simulink model "model_2springs_with_PSnum"  (R2023a)
settings: Solver=ode4  StartTime=0.0  StopTime=model.tmax  FixedStep=model.dt  RelTol=1e-3
values from neighbouring files (symbols this model uses):
  element : value not decoded    [Elem9_L5_NL4.sldd]
  model : value not decoded    [Elem9_L5_NL4.sldd]
settings Model: DataDictionary=model_2springs.sldd  Creator=glenn  LastModifiedBy=glenn
settings DataIOCC: SaveState=on
settings DebuggingCC: AlgebraicLoopMsg=none

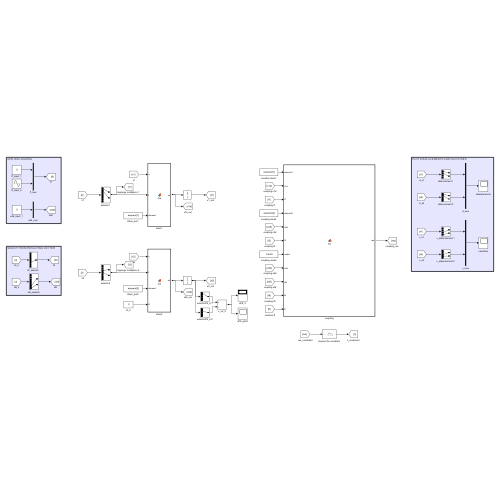
[thumbnail: Simulink's stored preview of the top-level diagram]
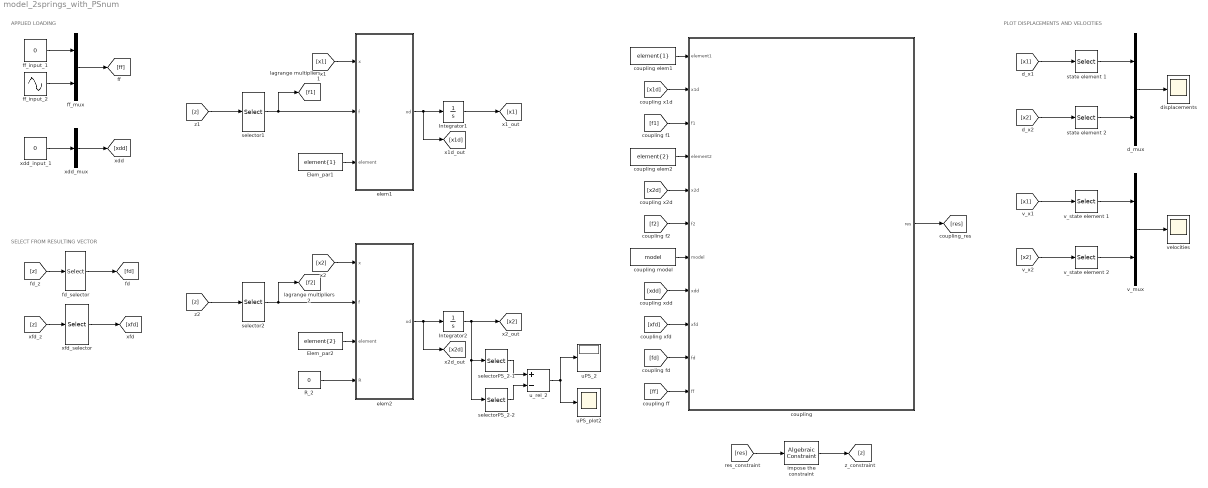
== system model_2springs_with_PSnum ==
  note: APPLIED LOADING
  note: SELECT FROM RESULTING VECTOR
  note: PLOT DISPLACEMENTS AND VELOCITIES
  Elem_par1 : Constant  Value=element{1}  OutDataTypeStr=Bus: ePar1
  Elem_par2 : Constant  Value=element{2}  OutDataTypeStr=Bus: ePar2
  Integrator1 : Integrator  InitialCondition=zeros(4,1)
  Integrator2 : Integrator  InitialCondition=zeros(5,1)
  R_2 : Constant  Value=0
  coupling : MATLAB Function  TreatAsAtomicUnit=on
  coupling elem1 : Constant  Value=element{1}  OutDataTypeStr=Bus: ePar1
  coupling elem2 : Constant  Value=element{2}  OutDataTypeStr=Bus: ePar2
  coupling model : Constant  Value=model  OutDataTypeStr=Bus: mPar
  d_mux : Mux  Inputs=2
  displacements : Scope
  elem1 : MATLAB Function  TreatAsAtomicUnit=on
  elem2 : MATLAB Function  TreatAsAtomicUnit=on
  fd_selector : Selector  InputPortWidth=7  IndexOptions=Index vector (dialog)  Indices=[5]  OutputSizes=1
  ff_input_1 : Constant  Value=0
  ff_input_2 : Sin  Amplitude=500  Frequency=6.2832  SampleTime=0
  ff_mux : Mux  Inputs=2
  impose the constraint : AlgebraicConstraint
  selector1 : Selector  InputPortWidth=7  IndexOptions=Index vector (dialog)  Indices="[1  2]"  OutputSizes=1
  selector2 : Selector  InputPortWidth=7  IndexOptions=Index vector (dialog)  Indices="[3  4]"  OutputSizes=1
  selectorPS_2-1 : Selector  InputPortWidth=5  IndexOptions=Index vector (dialog)  Indices=1  OutputSizes=1
  selectorPS_2-2 : Selector  InputPortWidth=5  IndexOptions=Index vector (dialog)  Indices=2  OutputSizes=1
  state element 1 : Selector  InputPortWidth=4  IndexOptions=Index vector (dialog)  Indices=[1 2]  OutputSizes=1
  state element 2 : Selector  InputPortWidth=5  IndexOptions=Index vector (dialog)  Indices=[1 2]  OutputSizes=1
  uPS_2 : Display
  uPS_plot2 : Scope
  u_rel_2 : Sum  Inputs=+-
  v_mux : Mux  Inputs=2
  v_state element 1 : Selector  InputPortWidth=4  IndexOptions=Index vector (dialog)  Indices=[3 4]  OutputSizes=1
  v_state element 2 : Selector  InputPortWidth=5  IndexOptions=Index vector (dialog)  Indices=[3 4]  OutputSizes=1
  velocities : Scope
  xdd_input_1 : Constant  Value=0
  xdd_mux : Mux  Inputs=1
  xfd_selector : Selector  InputPortWidth=7  IndexOptions=Index vector (dialog)  Indices="[6  7]"  OutputSizes=1
  wires:
  ff_input_1/1 -> ff_mux/1
  ff_input_2/1 -> ff_mux/2
  ff_mux/1 -> [ff]
  xdd_input_1/1 -> xdd_mux/1
  xdd_mux/1 -> [xdd]
  [z] -> fd_selector/1
  fd_selector/1 -> [fd]
  [z] -> xfd_selector/1
  xfd_selector/1 -> [xfd]
  [res] -> impose the constraint/1
  impose the constraint/1 -> [z]
  [x1] -> elem1/1(x)
  selector1/1 -> elem1/2(f), [f1]
  [z] -> selector1/1
  Elem_par1/1 -> elem1/3(element)
  elem1/1(xd) -> Integrator1/1, [x1d]
  Integrator1/1 -> [x1]
  coupling elem1/1 -> coupling/1(element1)
  [x1d] -> coupling/2(x1d)
  [f1] -> coupling/3(f1)
  [x2] -> elem2/1(x)
  selector2/1 -> elem2/2(f), [f2]
  [z] -> selector2/1
  Elem_par2/1 -> elem2/3(element)
  elem2/1(xd) -> Integrator2/1, [x2d]
  Integrator2/1 -> selectorPS_2-1/1, selectorPS_2-2/1, [x2]
  coupling elem2/1 -> coupling/4(element2)
  [x2d] -> coupling/5(x2d)
  [f2] -> coupling/6(f2)
  R_2/1 -> elem2/4(R)
  selectorPS_2-1/1 -> u_rel_2/1
  selectorPS_2-2/1 -> u_rel_2/2
  u_rel_2/1 -> uPS_2/1, uPS_plot2/1
  coupling model/1 -> coupling/7(model)
  [xdd] -> coupling/8(xdd)
  [xfd] -> coupling/9(xfd)
  [fd] -> coupling/10(fd)
  [ff] -> coupling/11(ff)
  coupling/1(res) -> [res]
  [x1] -> state element 1/1
  state element 1/1 -> d_mux/1
  [x2] -> state element 2/1
  state element 2/1 -> d_mux/2
  d_mux/1 -> displacements/1
  [x1] -> v_state element 1/1
  v_state element 1/1 -> v_mux/1
  [x2] -> v_state element 2/1
  v_state element 2/1 -> v_mux/2
  v_mux/1 -> velocities/1

== matlab function model_2springs_with_PSnum/elem2 ==
  data: x input; xd output; f input; element input; R input
function xd = fcn(x,f,element,R)

R = R_boucwen(x, element);
xd = element.M \ (element.B*f - R);

end

== matlab function model_2springs_with_PSnum/elem1 ==
  data: x input; xd output; f input; element input
function xd = fcn(x,f,element)

xd = element.M \ (element.B*f - R_linear(x,element));

end

== matlab function model_2springs_with_PSnum/coupling ==
  data: element1 input; res output; x1d input; f1 input; element2 input; x2d input; f2 input; model input; xdd input; xfd input; fd input; ff input
function res = fcn(element1,x1d,f1,element2,x2d,f2,model,xdd,xfd,fd,ff)

% Equilibrium
epsilon_B = element1.Bbar * f1 + element2.Bbar * f2 + model.Bbar_f * ff + model.Bbar_d * fd;

% Compatibility
epsilon_G = [
[element1.G_f; element1.G_d] * x1d + blkdiag(element1.Gbar_f, element1.Gbar_d) * [xfd; xdd] ;
element2.G_f * x2d + element2.Gbar_f * xfd ;
];

% Residuals
res = [epsilon_B; epsilon_G];

end
